simulink model "SwitchTest"  (R2019a)
settings: Solver=VariableStepAuto  StartTime=0.0  StopTime=10.0  RelTol=1e-3
undefined symbols (not defined in the file): constValue
settings Model: Creator=Safet  LastModifiedBy=Safet

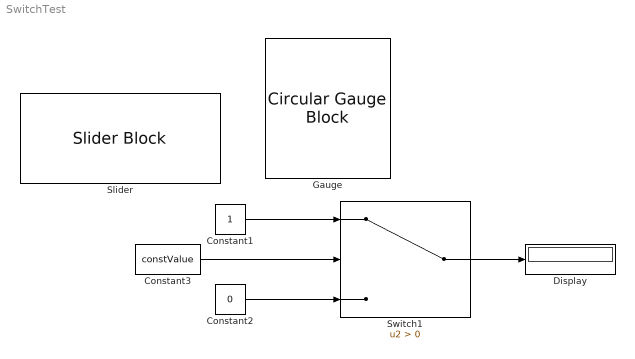
== system SwitchTest ==
  Constant1 : Constant
  Constant2 : Constant  Value=0
  Constant3 : Constant  Value=constValue
  Display : Display
  Gauge : CircularGaugeBlock  ScaleMin=-100
  Slider : SliderBlock  ScaleMin=-100
  Switch1 : Switch  Criteria=u2 > Threshold
  wires:
  Switch1/1 -> Display/1
  Constant2/1 -> Switch1/3
  Constant1/1 -> Switch1/1
  Constant3/1 -> Switch1/2
